simulink model "multiplexer"  (R2014a)
settings: Solver=ode45  StartTime=0.0  StopTime=10.0  RelTol=1e-3
settings Model: Creator=whitaker.an  LastModifiedBy=you.r
settings OptimizationCC: SimCompilerOptimization=off
settings DebuggingCC: MergeDetectMultiDrivingBlocksExec=error  FrameProcessingCompatibilityMsg=error
settings RTWCC: RTWCompilerOptimization=off
settings ConfigComp: CovMetricSettings=dw  CovHtmlReporting=on  CovSaveCumulativeToWorkspaceVar=on  CovSaveSingleToWorkspaceVar=on  CovModelRefEnable=Off  CovExternalEMLEnable=off  CovSFcnEnable=off

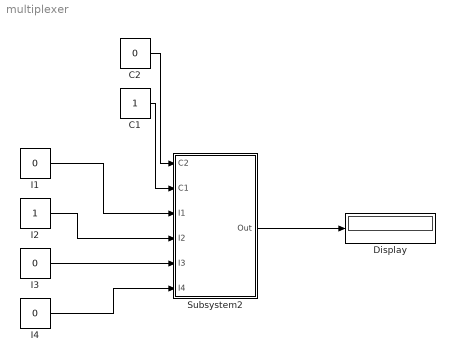
== system multiplexer ==
  C1 : Constant  OutDataTypeStr=boolean  SampleTime=1
  C2 : Constant  Value=0  OutDataTypeStr=boolean  SampleTime=1
  Display : Display
  I1 : Constant  Value=0  OutDataTypeStr=boolean  SampleTime=1
  I2 : Constant  OutDataTypeStr=boolean  SampleTime=1
  I3 : Constant  Value=0  OutDataTypeStr=boolean  SampleTime=1
  I4 : Constant  Value=0  OutDataTypeStr=boolean  SampleTime=1
  Subsystem2 : Subsystem
  wires:
  C2/1 -> Subsystem2/1(C2)
  C1/1 -> Subsystem2/2(C1)
  I1/1 -> Subsystem2/3(I1)
  I2/1 -> Subsystem2/4(I2)
  I3/1 -> Subsystem2/5(I3)
  I4/1 -> Subsystem2/6(I4)
  Subsystem2/1(Out) -> Display/1

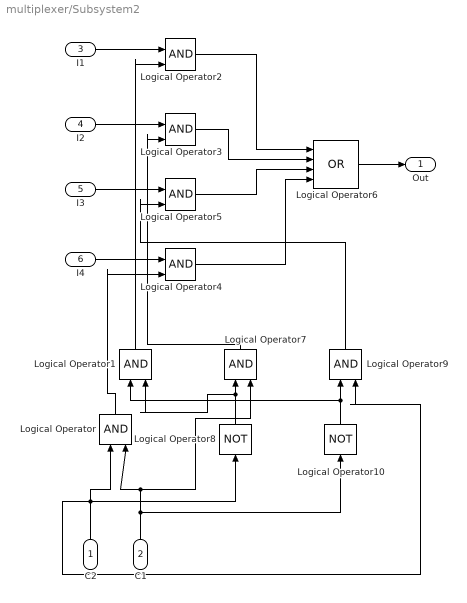
== system multiplexer/Subsystem2 ==
  C2 : Inport
  C1 : Inport  Port=2
  I1 : Inport  Port=3
  I2 : Inport  Port=4
  I3 : Inport  Port=5
  I4 : Inport  Port=6
  Logical Operator{,1..5,7,9} (8 alike) : Logic  IconShape=distinctive  AllPortsSameDT=off  OutDataTypeStr=boolean
  Logical Operator10 : Logic  Operator=NOT  IconShape=distinctive  AllPortsSameDT=off  OutDataTypeStr=boolean
  Logical Operator6 : Logic  Operator=OR  Inputs=4  IconShape=distinctive  AllPortsSameDT=off  OutDataTypeStr=boolean
  Logical Operator8 : Logic  Operator=NOT  IconShape=distinctive  AllPortsSameDT=off  OutDataTypeStr=boolean
  Out : Outport
  wires:
  I1/1 -> Logical Operator2/1
  I3/1 -> Logical Operator5/1
  Logical Operator4/1 -> Logical Operator6/4
  Logical Operator3/1 -> Logical Operator6/2
  C1/1 -> Logical Operator10/1, Logical Operator/2, Logical Operator7/2
  C2/1 -> Logical Operator9/2, Logical Operator/1, Logical Operator8/1
  Logical Operator10/1 -> Logical Operator1/1, Logical Operator9/1
  Logical Operator/1 -> Logical Operator4/2
  Logical Operator7/1 -> Logical Operator3/2
  I2/1 -> Logical Operator3/1
  Logical Operator2/1 -> Logical Operator6/1
  Logical Operator9/1 -> Logical Operator5/2
  I4/1 -> Logical Operator4/1
  Logical Operator5/1 -> Logical Operator6/3
  Logical Operator6/1 -> Out/1
  Logical Operator8/1 -> Logical Operator1/2, Logical Operator7/1
  Logical Operator1/1 -> Logical Operator2/2
